simulink model "fourth_1"  (R2021b)
settings: Solver=VariableStepAuto  StartTime=0.0  StopTime=10.0  RelTol=1e-3
settings Model: DataDictionary=my_k.sldd  Creator=fredric  LastModifiedBy=fredric

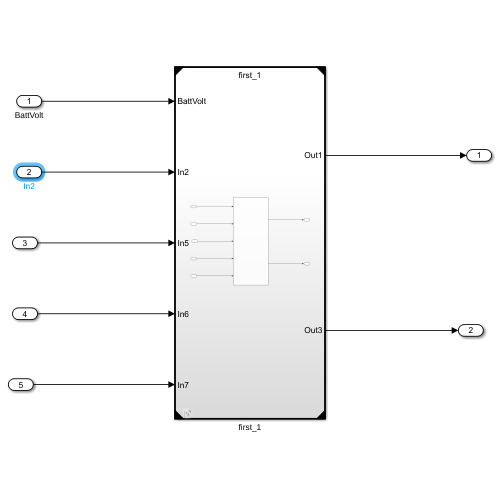
[thumbnail: Simulink's stored preview of the top-level diagram]
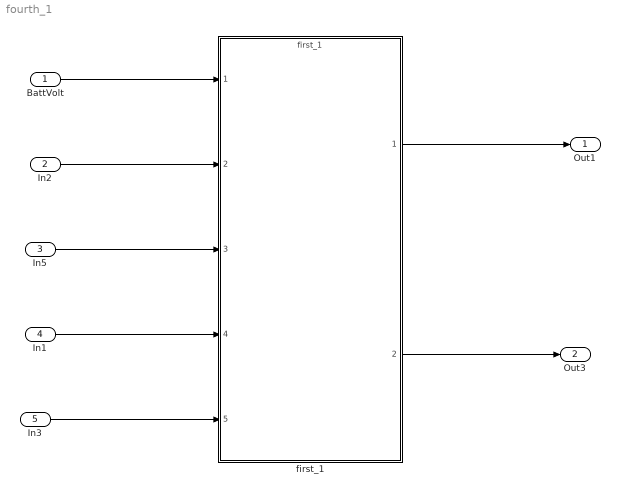
== system fourth_1 ==
  BattVolt : Inport
  In2 : Inport  Port=2
  In5 : Inport  Port=3
  In1 : Inport  Port=4
  In3 : Inport  Port=5
  first_1 : ModelReference  ModelNameDialog=first_1  ModelReferenceVersion=1.3
  Out1 : Outport
  Out3 : Outport  Port=2
  wires:
  BattVolt/1 -> first_1/1
  In2/1 -> first_1/2
  first_1/1 -> Out1/1
  In5/1 -> first_1/3
  In1/1 -> first_1/4
  In3/1 -> first_1/5
  first_1/2 -> Out3/1
